simulink model "CSE1_HIL_full16_caseB"  (R2018b)
settings: Solver=VariableStepAuto  StartTime=0.0  StopTime=500  MaxStep=10e-3  RelTol=1e-3
libraries: aerolibutil x1
settings Model: Creator=einarsu  LastModifiedBy=martin
settings OptimizationCC: LifeSpan=inf
settings DebuggingCC: SFExecutionAtInitializationDiag=none
settings SFSimCC: SimUseLocalCustomCode=off
settings RTWCC: RTWUseLocalCustomCode=off
settings CodeAppCC: StateflowObjectComments=on

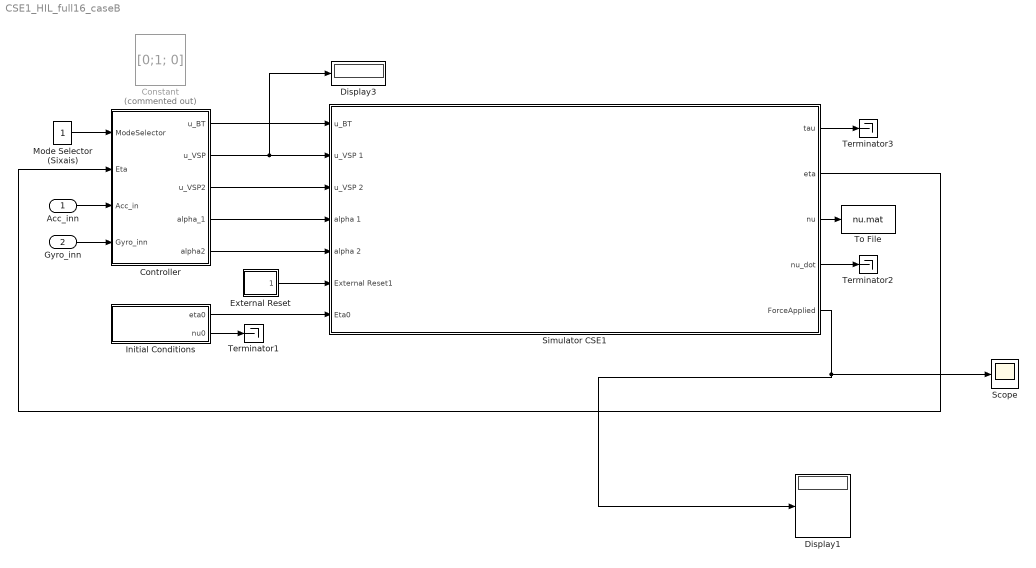
== system CSE1_HIL_full16_caseB ==
  Acc_inn : Inport
  Gyro_inn : Inport  Port=2
  Constant : Constant  Commented=on  Value=[0;1; 0]
  Controller : Subsystem
  Display1 : Display
  Display3 : Display
  External Reset : Subsystem
  "Initial Conditions " : Subsystem
  Mode Selector (Sixais) : Constant
  Scope : Scope
  Simulator CSE1 : Subsystem
  Terminator1 : Terminator
  Terminator2 : Terminator
  Terminator3 : Terminator
  To File : ToFile  Filename=nu.mat  MatrixName=nu
  wires:
  Controller/1(u_BT) -> Simulator CSE1/1(u_BT)
  Controller/4(alpha_1) -> Simulator CSE1/4(alpha 1)
  Controller/2(u_VSP) -> Display3/1, Simulator CSE1/2(u_VSP 1)
  Controller/5(alpha2) -> Simulator CSE1/5(alpha 2)
  Controller/3("u_VSP2 ") -> Simulator CSE1/3(u_VSP 2)
  External Reset/1(Out1) -> Simulator CSE1/6(External Reset1)
  "Initial Conditions "/1(eta0) -> Simulator CSE1/7(Eta0)
  Mode Selector (Sixais)/1 -> Controller/1(ModeSelector)
  Simulator CSE1/2(eta) -> Controller/2(Eta)
  Acc_inn/1 -> Controller/3(Acc_in)
  Gyro_inn/1 -> Controller/4(Gyro_inn)
  Simulator CSE1/5(ForceApplied) -> Scope/1, Display1/1
  "Initial Conditions "/2(nu0) -> Terminator1/1
  Simulator CSE1/4(nu_dot) -> Terminator2/1
  Simulator CSE1/3(nu) -> To File/1
  Simulator CSE1/1(tau) -> Terminator3/1

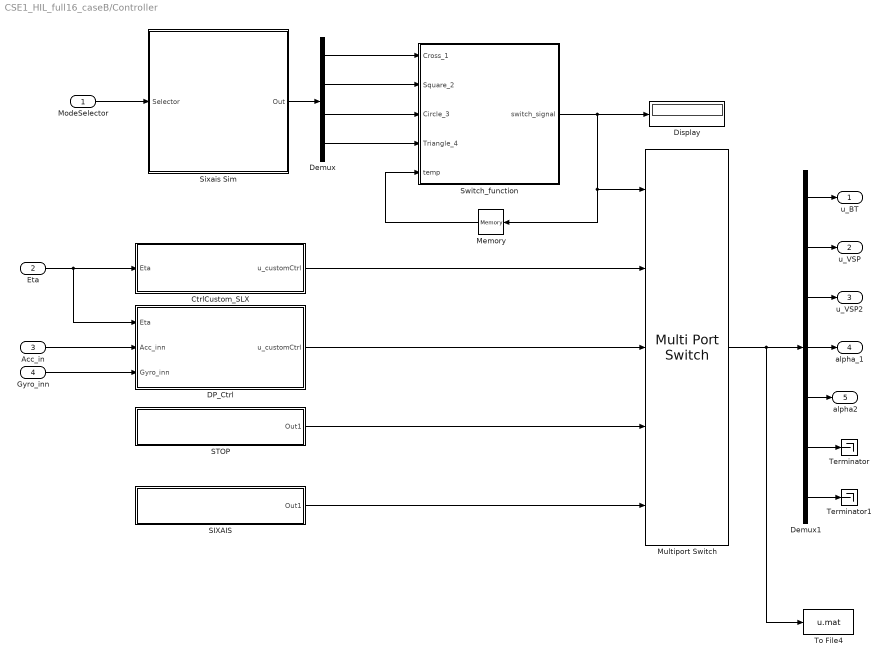
== system CSE1_HIL_full16_caseB/Controller ==
  ModeSelector : Inport
  Eta : Inport  Port=2
  Acc_in : Inport  Port=3
  Gyro_inn : Inport  Port=4
  CtrlCustom_SLX : Subsystem
  DP_Ctrl : Subsystem
  Demux : Demux
  Demux1 : Demux  Outputs=7
  Display : Display
  Memory : Memory  InitialCondition=4
  Multiport Switch : MultiPortSwitch  Inputs=4
  SIXAIS : Subsystem
  STOP : Subsystem
  Sixais Sim : MATLAB Function  TreatAsAtomicUnit=on
  Switch_function : MATLAB Function  TreatAsAtomicUnit=on
  Terminator : Terminator
  Terminator1 : Terminator
  To File4 : ToFile  Filename=u.mat  MatrixName=u
  u_BT : Outport
  u_VSP : Outport  Port=2
  "u_VSP2 " : Outport  Port=3
  alpha_1 : Outport  Port=4
  alpha2 : Outport  Port=5
  wires:
  Memory/1 -> Switch_function/5(temp)
  CtrlCustom_SLX/1(u_customCtrl) -> Multiport Switch/2
  Demux/1 -> Switch_function/1(Cross_1)
  Demux/2 -> Switch_function/2(Square_2)
  Demux/3 -> Switch_function/3(Circle_3)
  Demux/4 -> Switch_function/4(Triangle_4)
  Sixais Sim/1(Out) -> Demux/1
  ModeSelector/1 -> Sixais Sim/1(Selector)
  STOP/1(Out1) -> Multiport Switch/4
  SIXAIS/1(Out1) -> Multiport Switch/5
  Eta/1 -> CtrlCustom_SLX/1(Eta), DP_Ctrl/1(Eta)
  Multiport Switch/1 -> To File4/1, Demux1/1
  Demux1/1 -> u_BT/1
  Demux1/2 -> u_VSP/1
  Demux1/3 -> "u_VSP2 "/1
  Demux1/4 -> alpha_1/1
  Demux1/5 -> alpha2/1
  Demux1/6 -> Terminator/1
  Demux1/7 -> Terminator1/1
  Acc_in/1 -> DP_Ctrl/2(Acc_inn)
  Gyro_inn/1 -> DP_Ctrl/3(Gyro_inn)
  DP_Ctrl/1(u_customCtrl) -> Multiport Switch/3
  Switch_function/1(switch_signal) -> Display/1, Memory/1, Multiport Switch/1

== system CSE1_HIL_full16_caseB/External Reset ==
  note: Most relevant for Real-Time Simulations...
  Constant : Constant  Value=0
  Out1 : Outport
  wires:
  Constant/1 -> Out1/1

== system CSE1_HIL_full16_caseB/Initial Conditions  ==
  Eta0 : Constant  Value=zeros(3,1)
  "V0 " : Constant  Value=zeros(3,1)
  eta0 : Outport
  nu0 : Outport  Port=2
  wires:
  "V0 "/1 -> nu0/1
  Eta0/1 -> eta0/1

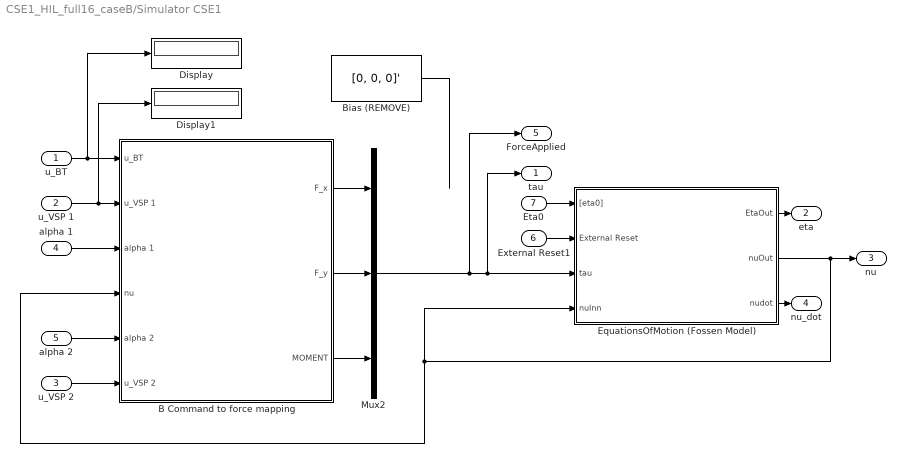
== system CSE1_HIL_full16_caseB/Simulator CSE1 ==
  u_BT : Inport
  u_VSP 1 : Inport  Port=2
  u_VSP 2 : Inport  Port=3
  alpha 1 : Inport  Port=4
  alpha 2 : Inport  Port=5
  External Reset1 : Inport  Port=6
  Eta0 : Inport  Port=7
  B Command to force mapping : Subsystem
  Bias (REMOVE) : Constant  Value=[0, 0, 0]'
  Display : Display
  Display1 : Display
  EquationsOfMotion (Fossen Model) : Subsystem
  Mux2 : Mux  Inputs=3
  tau : Outport
  eta : Outport  Port=2
  nu : Outport  Port=3
  nu_dot : Outport  Port=4
  ForceApplied : Outport  Port=5
  wires:
  alpha 2/1 -> B Command to force mapping/5(alpha 2)
  B Command to force mapping/2("F_y ") -> Mux2/2
  B Command to force mapping/1(F_x) -> Mux2/1
  u_VSP 1/1 -> Display1/1, B Command to force mapping/2(u_VSP 1)
  alpha 1/1 -> B Command to force mapping/3(alpha 1)
  u_BT/1 -> Display/1, B Command to force mapping/1(u_BT)
  u_VSP 2/1 -> B Command to force mapping/6(u_VSP 2)
  EquationsOfMotion (Fossen Model)/2(nuOut) -> B Command to force mapping/4(nu), EquationsOfMotion (Fossen Model)/4(nuInn), nu/1
  Eta0/1 -> EquationsOfMotion (Fossen Model)/1("[eta0] ")
  External Reset1/1 -> EquationsOfMotion (Fossen Model)/2(External Reset)
  EquationsOfMotion (Fossen Model)/1(EtaOut) -> eta/1
  EquationsOfMotion (Fossen Model)/3(nudot) -> nu_dot/1
  B Command to force mapping/3("MOMENT ") -> Mux2/3
  Mux2/1 -> ForceApplied/1, EquationsOfMotion (Fossen Model)/3(tau), tau/1
  Bias (REMOVE)/1 -> ?

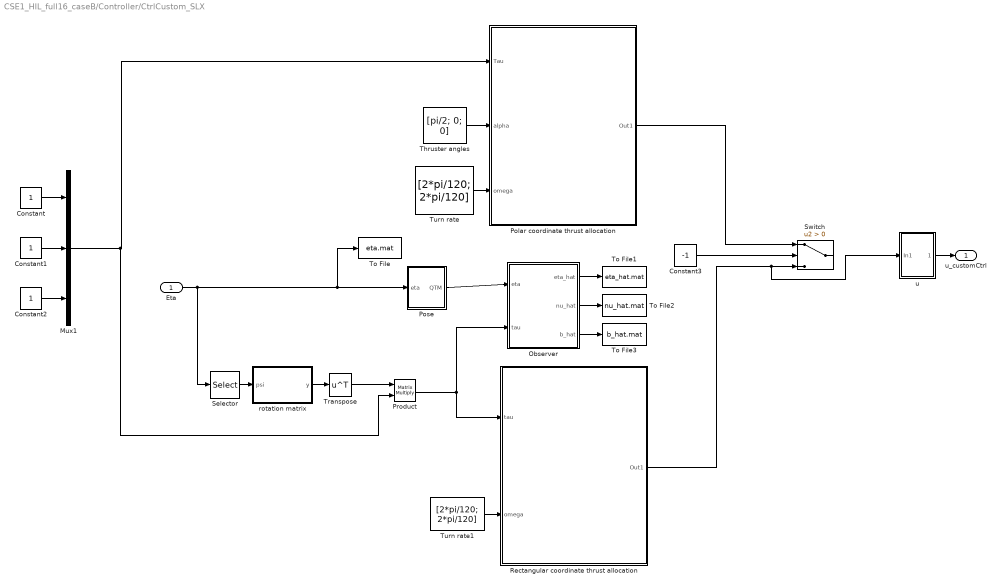
== system CSE1_HIL_full16_caseB/Controller/CtrlCustom_SLX ==
  Eta : Inport
  Constant : Constant
  Constant1 : Constant
  Constant2 : Constant
  Constant3 : Constant  Value=-1
  Mux1 : Mux  Inputs=3
  Observer : Subsystem
  Polar coordinate thrust allocation : Subsystem
  Pose : Subsystem
  Product : Product  Multiplication=Matrix(*)
  Rectangular coordinate thrust allocation : Subsystem
  Selector : Selector  InputPortWidth=3  IndexOptions=Index vector (dialog)  Indices=[3]  OutputSizes=1
  Switch : Switch  Criteria=u2 > Threshold
  Thruster angles : Constant  Value=[pi/2; 0; 0]  VectorParams1D=off
  To File : ToFile  Filename=eta.mat  MatrixName=eta
  To File1 : ToFile  Filename=eta_hat.mat  MatrixName=eta_hat
  To File2 : ToFile  Filename=nu_hat.mat  MatrixName=nu_hat
  To File3 : ToFile  Filename=b_hat.mat  MatrixName=b_hat
  Transpose : Math  Operator=transpose  SaturateOnIntegerOverflow=on
  Turn rate : Constant  Value=[2*pi/120; 2*pi/120]  VectorParams1D=off
  Turn rate1 : Constant  Value=[2*pi/120; 2*pi/120]  VectorParams1D=off
  rotation matrix : MATLAB Function  TreatAsAtomicUnit=on
  u : Subsystem
  u_customCtrl : Outport
  wires:
  Rectangular coordinate thrust allocation/1(Out1) -> u/1(In1), Switch/3
  Turn rate1/1 -> Rectangular coordinate thrust allocation/2("omega ")
  Turn rate/1 -> Polar coordinate thrust allocation/3("omega ")
  Thruster angles/1 -> Polar coordinate thrust allocation/2(alpha)
  Eta/1 -> To File/1, Pose/1(eta), Selector/1
  u/1(Out1) -> u_customCtrl/1
  Polar coordinate thrust allocation/1(Out1) -> Switch/1
  Constant2/1 -> Mux1/3
  Constant1/1 -> Mux1/2
  Constant/1 -> Mux1/1
  Pose/1(QTM) -> Observer/1(eta)
  Mux1/1 -> Product/2, Polar coordinate thrust allocation/1(Tau)
  Observer/1(eta_hat) -> To File1/1
  Observer/2("nu_hat ") -> To File2/1
  Observer/3(b_hat) -> To File3/1
  Constant3/1 -> Switch/2
  Selector/1 -> rotation matrix/1(psi)
  rotation matrix/1(y) -> Transpose/1
  Product/1 -> Observer/2(tau), Rectangular coordinate thrust allocation/1(tau)
  Transpose/1 -> Product/1

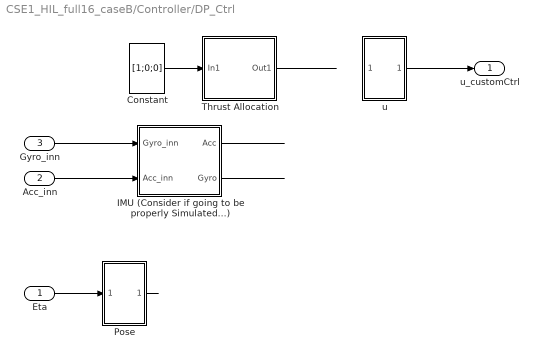
== system CSE1_HIL_full16_caseB/Controller/DP_Ctrl ==
  Eta : Inport
  Acc_inn : Inport  Port=2
  Gyro_inn : Inport  Port=3
  Constant : Constant  Value=[1;0;0]
  IMU (Consider if going to be properly Simulated...) : Subsystem
  Pose : Subsystem
  "Thrust Allocation " : Subsystem
  u : Subsystem
  u_customCtrl : Outport
  wires:
  Pose/1(QTM) -> ?
  Gyro_inn/1 -> IMU (Consider if going to be properly Simulated...)/1(Gyro_inn)
  Acc_inn/1 -> IMU (Consider if going to be properly Simulated...)/2(Acc_inn)
  Eta/1 -> Pose/1(eta)
  u/1(Out1) -> u_customCtrl/1
  IMU (Consider if going to be properly Simulated...)/2(Gyro) -> ?
  IMU (Consider if going to be properly Simulated...)/1(Acc) -> ?
  Constant/1 -> "Thrust Allocation "/1(In1)
  "Thrust Allocation "/1(Out1) -> ?

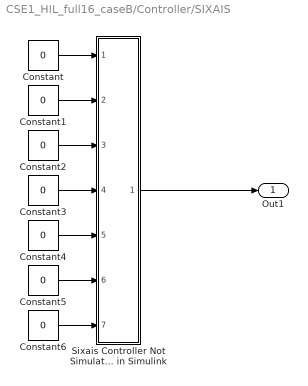
== system CSE1_HIL_full16_caseB/Controller/SIXAIS ==
  Constant{,1..6} (7 alike) : Constant  Value=0
  Sixais Controller Not Simulated in Simulink : Subsystem
  Out1 : Outport
  wires:
  Constant/1 -> Sixais Controller Not Simulated in Simulink/1(In1)
  Constant1/1 -> Sixais Controller Not Simulated in Simulink/2(In2)
  Constant2/1 -> Sixais Controller Not Simulated in Simulink/3(In3)
  Constant3/1 -> Sixais Controller Not Simulated in Simulink/4(In4)
  Constant4/1 -> Sixais Controller Not Simulated in Simulink/5(In5)
  Constant5/1 -> Sixais Controller Not Simulated in Simulink/6(In6)
  Constant6/1 -> Sixais Controller Not Simulated in Simulink/7(In7)
  Sixais Controller Not Simulated in Simulink/1(Out1) -> Out1/1

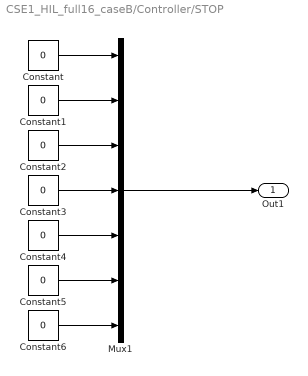
== system CSE1_HIL_full16_caseB/Controller/STOP ==
  Constant{,1..6} (7 alike) : Constant  Value=0
  Mux1 : Mux  Inputs=7
  Out1 : Outport
  wires:
  Mux1/1 -> Out1/1
  Constant/1 -> Mux1/1
  Constant1/1 -> Mux1/2
  Constant2/1 -> Mux1/3
  Constant3/1 -> Mux1/4
  Constant4/1 -> Mux1/5
  Constant5/1 -> Mux1/6
  Constant6/1 -> Mux1/7

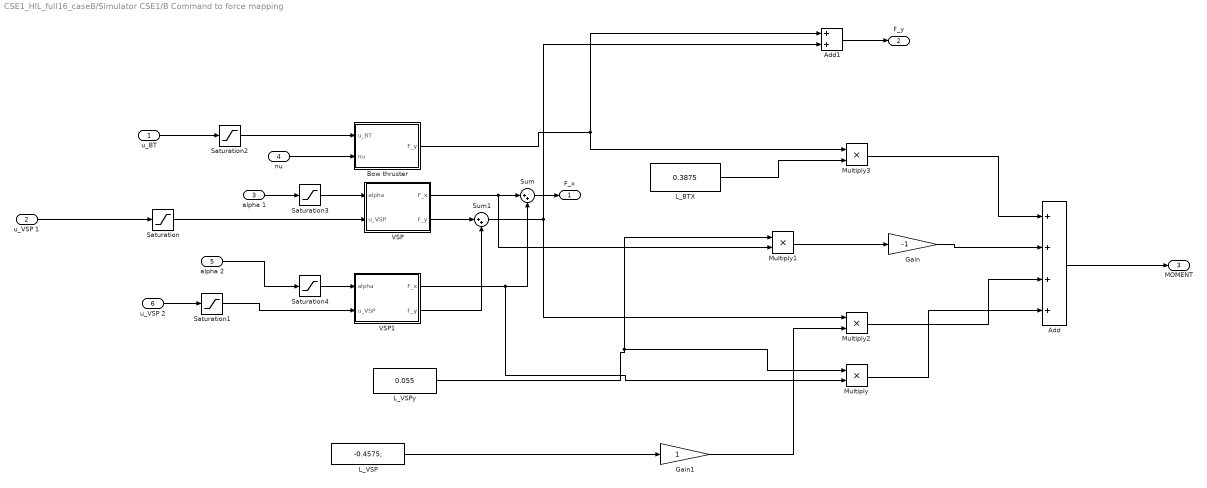
== system CSE1_HIL_full16_caseB/Simulator CSE1/B Command to force mapping ==
  u_BT : Inport
  u_VSP 1 : Inport  Port=2
  alpha 1 : Inport  Port=3
  nu : Inport  Port=4
  alpha 2 : Inport  Port=5
  u_VSP 2 : Inport  Port=6
  Add : Sum  Inputs=++++
  Add1 : Sum
  Bow thruster : MATLAB Function  TreatAsAtomicUnit=on
  Gain : Gain  Gain=-1
  Gain1 : Gain
  L_BTX : Constant  Value=0.3875
  L_VSP : Constant  Value=-0.4575;
  L_VSPy : Constant  Value=0.055
  Multiply{,1..3} (4 alike) : Product
  Saturation : Saturate  UpperLimit=1  LowerLimit=0
  Saturation1 : Saturate  UpperLimit=1  LowerLimit=0
  Saturation2 : Saturate  UpperLimit=1  LowerLimit=-1
  Saturation3 : Saturate  UpperLimit=pi  LowerLimit=-pi
  Saturation4 : Saturate  UpperLimit=pi  LowerLimit=-pi
  Sum : Sum  Inputs=|++
  Sum1 : Sum  Inputs=|++
  VSP : MATLAB Function  TreatAsAtomicUnit=on
  VSP1 : MATLAB Function  TreatAsAtomicUnit=on
  F_x : Outport
  "F_y " : Outport  Port=2
  "MOMENT " : Outport  Port=3
  wires:
  alpha 1/1 -> Saturation3/1
  nu/1 -> Bow thruster/2(nu)
  Bow thruster/1(F_y) -> Add1/1, Multiply3/1
  VSP/2(F_y) -> Sum1/1
  Sum1/1 -> Add1/2, Multiply2/1
  VSP1/2(F_y) -> Sum1/2
  VSP1/1(F_x) -> Multiply/2, Sum/2
  VSP/1(F_x) -> Multiply1/2, Sum/1
  Sum/1 -> F_x/1
  alpha 2/1 -> Saturation4/1
  u_VSP 2/1 -> Saturation1/1
  L_VSP/1 -> Gain1/1
  L_BTX/1 -> Multiply3/2
  L_VSPy/1 -> Multiply/1, Multiply1/1
  Multiply3/1 -> Add/1
  Multiply1/1 -> Gain/1
  Multiply2/1 -> Add/3
  Multiply/1 -> Add/4
  Add/1 -> "MOMENT "/1
  Gain/1 -> Add/2
  Gain1/1 -> Multiply2/2
  Add1/1 -> "F_y "/1
  Saturation/1 -> VSP/2(u_VSP)
  Saturation1/1 -> VSP1/2(u_VSP)
  u_BT/1 -> Saturation2/1
  u_VSP 1/1 -> Saturation/1
  Saturation2/1 -> Bow thruster/1(u_BT)
  Saturation3/1 -> VSP/1(alpha)
  Saturation4/1 -> VSP1/1(alpha)

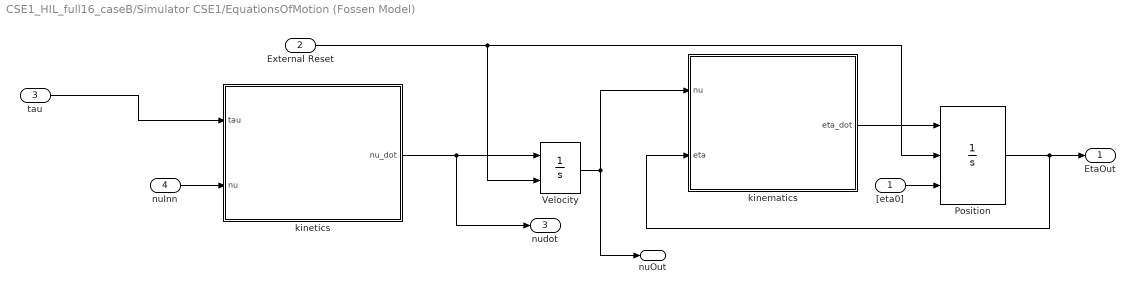
== system CSE1_HIL_full16_caseB/Simulator CSE1/EquationsOfMotion (Fossen Model) ==
  "[eta0] " : Inport
  External Reset : Inport  Port=2
  tau : Inport  Port=3
  nuInn : Inport  Port=4
  Position : Integrator  ExternalReset=either  InitialConditionSource=external  InitialCondition=[0 0 0]'
  Velocity : Integrator  ExternalReset=either  InitialCondition=[0 0 0]'
  kinematics : MATLAB Function  TreatAsAtomicUnit=on
  kinetics : MATLAB Function  TreatAsAtomicUnit=on
  EtaOut : Outport
  nuOut : Outport  Port=2
  nudot : Outport  Port=3
  wires:
  tau/1 -> kinetics/1(tau)
  Position/1 -> kinematics/2(eta), EtaOut/1
  "[eta0] "/1 -> Position/3
  nuInn/1 -> kinetics/2(nu)
  kinematics/1(eta_dot) -> Position/1
  Velocity/1 -> kinematics/1(nu), nuOut/1
  kinetics/1(nu_dot) -> nudot/1, Velocity/1
  External Reset/1 -> Position/2, Velocity/2

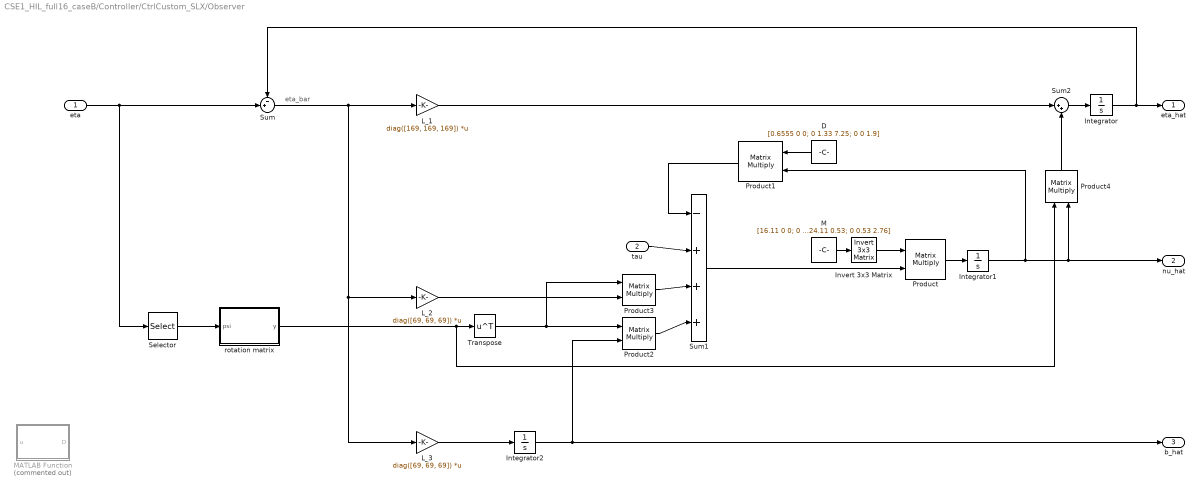
== system CSE1_HIL_full16_caseB/Controller/CtrlCustom_SLX/Observer ==
  note: eta_bar
  eta : Inport
  tau : Inport  Port=2
  D : Constant  Value=[0.6555 0 0; 0 1.33 7.25; 0 0 1.9]
  Integrator : Integrator  InitialCondition=[0 0 0]'
  Integrator1 : Integrator  InitialCondition=[0 0 0]'
  Integrator2 : Integrator
  Invert 3x3 Matrix : aerolibutil/Invert  3x3 Matrix
  L_1 : Gain  Gain=diag([169, 169, 169])  Multiplication=Matrix(K*u)
  L_2 : Gain  Gain=diag([69, 69, 69])  Multiplication=Matrix(K*u)
  L_3 : Gain  Gain=diag([69, 69, 69])  Multiplication=Matrix(K*u)
  M : Constant  Value=[16.11 0 0; 0 24.11 0.53; 0 0.53 2.76]
  MATLAB Function : MATLAB Function  Commented=on  TreatAsAtomicUnit=on
  Product{,1..4} (5 alike) : Product  Multiplication=Matrix(*)
  Selector : Selector  InputPortWidth=3  IndexOptions=Index vector (dialog)  Indices=[3]  OutputSizes=1
  Sum : Sum  Inputs=-+|
  Sum1 : Sum  Inputs=-|+|+|+
  Sum2 : Sum  Inputs=|++
  Transpose : Math  Operator=transpose  SaturateOnIntegerOverflow=on
  rotation matrix : MATLAB Function  TreatAsAtomicUnit=on
  eta_hat : Outport
  "nu_hat " : Outport  Port=2
  b_hat : Outport  Port=3
  wires:
  Sum/1 -> L_3/1, L_2/1, L_1/1
  eta/1 -> Selector/1, Sum/2
  Selector/1 -> rotation matrix/1(psi)
  Integrator/1 -> eta_hat/1, Sum/1
  Invert 3x3 Matrix/1 -> Product/1
  M/1 -> Invert 3x3 Matrix/1
  D/1 -> Product1/1
  Product1/1 -> Sum1/1
  rotation matrix/1(y) -> Product4/1, Transpose/1
  Transpose/1 -> Product3/1, Product2/1
  L_2/1 -> Product3/2
  Sum1/1 -> Product/2
  Product/1 -> Integrator1/1
  L_1/1 -> Sum2/1
  Product4/1 -> Sum2/2
  Sum2/1 -> Integrator/1
  Integrator1/1 -> Product1/2, Product4/2, "nu_hat "/1
  L_3/1 -> Integrator2/1
  Integrator2/1 -> Product2/2, b_hat/1
  Product2/1 -> Sum1/4
  Product3/1 -> Sum1/3
  tau/1 -> Sum1/2

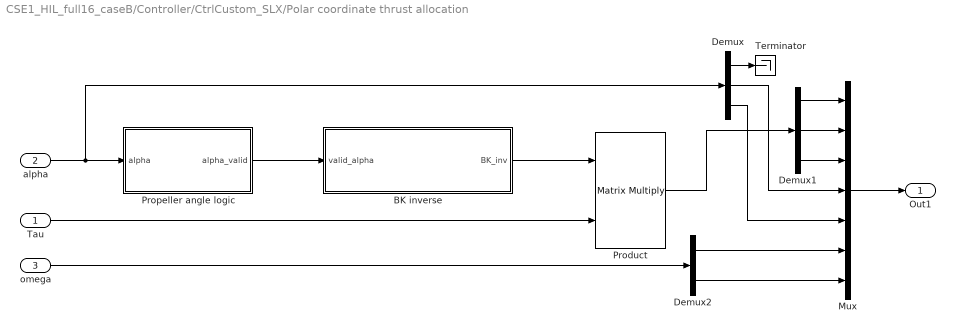
== system CSE1_HIL_full16_caseB/Controller/CtrlCustom_SLX/Polar coordinate thrust allocation ==
  Tau : Inport
  alpha : Inport  Port=2
  "omega " : Inport  Port=3
  "BK inverse " : MATLAB Function  TreatAsAtomicUnit=on
  Demux : Demux  Outputs=3
  Demux1 : Demux  Outputs=3
  Demux2 : Demux  Outputs=2
  Mux : Mux  Inputs=7
  Product : Product  Multiplication=Matrix(*)
  Propeller angle logic : MATLAB Function  TreatAsAtomicUnit=on
  Terminator : Terminator
  Out1 : Outport
  wires:
  Demux2/2 -> Mux/7
  Demux2/1 -> Mux/6
  Product/1 -> Demux1/1
  Demux1/3 -> Mux/3
  Demux1/2 -> Mux/2
  Demux1/1 -> Mux/1
  Demux/3 -> Mux/5
  Demux/2 -> Mux/4
  Demux/1 -> Terminator/1
  Mux/1 -> Out1/1
  "omega "/1 -> Demux2/1
  Tau/1 -> Product/2
  "BK inverse "/1(BK_inv) -> Product/1
  Propeller angle logic/1(alpha_valid) -> "BK inverse "/1(valid_alpha)
  alpha/1 -> Propeller angle logic/1(alpha), Demux/1

== system CSE1_HIL_full16_caseB/Controller/CtrlCustom_SLX/Pose ==
  eta : Inport
  Demux : Demux  Outputs=3
  Mux : Mux  Inputs=3
  QTM : Outport
  wires:
  eta/1 -> Demux/1
  Mux/1 -> QTM/1
  Demux/1 -> Mux/1  "x_m"
  Demux/3 -> Mux/3  "psi_m"
  Demux/2 -> Mux/2  "y_m"

== system CSE1_HIL_full16_caseB/Controller/CtrlCustom_SLX/Rectangular coordinate thrust allocation ==
  tau : Inport
  "omega " : Inport  Port=2
  Demux : Demux  Outputs=5
  Demux1 : Demux  Outputs=2
  MATLAB Function : MATLAB Function  TreatAsAtomicUnit=on
  Mux : Mux  Inputs=7
  Selector : Selector  InputPortWidth=5  IndexOptions=Index vector (dialog)  Indices=[3 1 2 4 5]  OutputSizes=1
  Out1 : Outport
  wires:
  Mux/1 -> Out1/1
  Demux1/1 -> Mux/6
  Demux1/2 -> Mux/7
  Demux/5 -> Mux/5
  Demux/4 -> Mux/4
  "omega "/1 -> Demux1/1
  MATLAB Function/1(u_ext) -> Selector/1
  tau/1 -> MATLAB Function/1(tau)
  Demux/1 -> Mux/1
  Demux/2 -> Mux/2
  Demux/3 -> Mux/3
  Selector/1 -> Demux/1

== system CSE1_HIL_full16_caseB/Controller/CtrlCustom_SLX/u ==
  In1 : Inport
  Demux1 : Demux  Outputs=7
  Mux : Mux  Inputs=7
  Saturation1 : Saturate  UpperLimit=1  LowerLimit=0
  Saturation11 : Saturate  UpperLimit=1  LowerLimit=0
  Saturation2 : Saturate  UpperLimit=1  LowerLimit=-1
  Out1 : Outport
  wires:
  Saturation1/1 -> Mux/3
  Saturation11/1 -> Mux/2
  Mux/1 -> Out1/1
  Demux1/7 -> Mux/7  "omega_VSP2"
  Demux1/6 -> Mux/6  "omega_VSP1"
  Demux1/5 -> Mux/5  "alpha_VSP2"
  Demux1/4 -> Mux/4  "alpha_VSP1"
  Demux1/3 -> Saturation1/1  "u_VSP2"
  Demux1/2 -> Saturation11/1  "u_VSP1"
  Demux1/1 -> Saturation2/1  "u_BT"
  In1/1 -> Demux1/1
  Saturation2/1 -> Mux/1

== system CSE1_HIL_full16_caseB/Controller/DP_Ctrl/IMU (Consider if going to be properly Simulated...) ==
  Gyro_inn : Inport
  Acc_inn : Inport  Port=2
  Demux : Demux  Outputs=3
  Demux1 : Demux  Outputs=3
  Mux : Mux  Inputs=3
  Mux2 : Mux  Inputs=3
  Acc : Outport
  Gyro : Outport  Port=2
  wires:
  Acc_inn/1 -> Demux1/1
  Gyro_inn/1 -> Demux/1
  Demux/1 -> Mux2/1
  Demux/2 -> Mux2/2
  Demux/3 -> Mux2/3
  Demux1/2 -> Mux/2
  Demux1/3 -> Mux/3
  Mux2/1 -> Gyro/1
  Demux1/1 -> Mux/1
  Mux/1 -> Acc/1

== system CSE1_HIL_full16_caseB/Controller/DP_Ctrl/Pose ==
  eta : Inport
  Demux : Demux  Outputs=3
  Mux : Mux  Inputs=3
  QTM : Outport
  wires:
  eta/1 -> Demux/1
  Mux/1 -> QTM/1
  Demux/1 -> Mux/1  "x_m"
  Demux/3 -> Mux/3  "psi_m"
  Demux/2 -> Mux/2  "y_m"

== system CSE1_HIL_full16_caseB/Controller/DP_Ctrl/Thrust Allocation  ==
  In1 : Inport
  THALOC (u->tau) : MATLAB Function  TreatAsAtomicUnit=on
  Out1 : Outport
  wires:
  In1/1 -> THALOC (u->tau)/1(u)
  THALOC (u->tau)/1(y) -> Out1/1

== system CSE1_HIL_full16_caseB/Controller/DP_Ctrl/u ==
  In1 : Inport
  Demux1 : Demux  Outputs=7
  Mux : Mux  Inputs=7
  Out1 : Outport
  wires:
  Mux/1 -> Out1/1
  Demux1/7 -> Mux/7  "omega_VSP2"
  Demux1/6 -> Mux/6  "omega_VSP1"
  Demux1/5 -> Mux/5  "alpha_VSP2"
  Demux1/4 -> Mux/4  "alpha_VSP1"
  Demux1/3 -> Mux/3  "u_VSP2"
  Demux1/2 -> Mux/2  "u_VSP1"
  Demux1/1 -> Mux/1  "u_BT"
  In1/1 -> Demux1/1

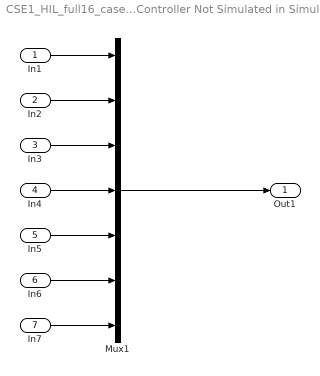
== system CSE1_HIL_full16_caseB/Controller/SIXAIS/Sixais Controller Not Simulated in Simulink ==
  In1 : Inport
  In2 : Inport  Port=2
  In3 : Inport  Port=3
  In4 : Inport  Port=4
  In5 : Inport  Port=5
  In6 : Inport  Port=6
  In7 : Inport  Port=7
  Mux1 : Mux  Inputs=7
  Out1 : Outport
  wires:
  In4/1 -> Mux1/4
  In5/1 -> Mux1/5
  In6/1 -> Mux1/6
  In3/1 -> Mux1/3
  In1/1 -> Mux1/1
  In2/1 -> Mux1/2
  Mux1/1 -> Out1/1
  In7/1 -> Mux1/7

== matlab function CSE1_HIL_full16_caseB/Simulator CSE1/EquationsOfMotion (Fossen Model)/kinematics ==
  data: nu input; eta_dot output; eta input
function eta_dot = CSE1_eta_dot(nu,eta)

psi = eta(3);

J = [cos(psi) -sin(psi) 0
     sin(psi) cos(psi)  0
     0        0         1];

eta_dot = J*nu;

== matlab function CSE1_HIL_full16_caseB/Simulator CSE1/EquationsOfMotion (Fossen Model)/kinetics ==
  data: tau input; nu_dot output; nu input
function nu_dot = CSE1_nu_dot(tau,nu)

u   = nu(1);
v   = nu(2);
r   = nu(3);

tau = [tau(1);tau(2);tau(3)];
%% MATRICES 
%changed m from 14.79 to 14.11

m    = 14.11;   I_z  =  1.7600;   x_g = 0.0375;       % x_g  =  0.0460; % Table B.1

%% Added mass
%changed Y_vd from -1.0 to -10.0
X_ud  =     -2.0;											% Table B.1
					Y_vd =      -10.0;	N_vd =    -0.0;		% Table B.1
					Y_rd =      -0.0;	N_rd =    -1.0;		% Table B.1

%% Total mass matrix
m_11 = m-X_ud;
m_22 = m-Y_vd;
m_23 = m*x_g-Y_rd;
m_32 = m*x_g-N_vd; % noted as Y_rd in handbook, but same value
m_33 = I_z-N_rd;

M    = [m_11 0    0
        0    m_22 m_23
        0    m_32 m_33];
	
%% Damping coefficients
% Comments at the end of the lines indicate the old values used.
X_u		= -0.6555;		X_v		= 0;
X_uu 	= 0.3545;		X_vv	= -2.443;
X_uuu 	= -3.787;		X_vvv	= 0;

						Y_v		= -1.33; 			Y_r		= -7.250; % Y_r
						Y_vv	= -2.776;			Y_rr	= -3.450; % Y_rr
						Y_vvv	= -64.91;			Y_rrr	= 0;
						
						Y_rv	= -0.805;			Y_vr	= -0.845; % Y_rv, Y_vr

						N_v		= 0;				N_r		= -1.900; % N_r
						N_vv	= -0.2088;			N_rr	= -0.750; % N_rr
						N_vvv	= 0;				N_rrr	= 0;
						
						N_rv	= 0.130;			N_vr	= 0.080; % N_rv, N_vr

%% Correolis matrix
c_13 = -(m-Y_vd)*v-(m*x_g-Y_rd)*r;
c_23 = (m-X_ud)*u;
C    = [0     0     c_13
        0     0     c_23
        -c_13 -c_23 0   ];

%% Assembly of the damping matrix
%should be abs(u), abs(v) some places, only positive values? 

d_11 = -X_u - X_uu*u - X_uuu*u^2;
d_22 = -Y_v - Y_vv*v - Y_vvv*v^2 - Y_rv*abs(r);
d_33 = -N_r - N_rr*abs(r) - N_rrr*r^2 - N_vr*abs(v); % using abs(r)

d_12 = -X_v - X_vv*v - X_vvv*v^2;
d_23 = -Y_r - Y_rr*abs(r) - Y_rrr*r^2 - Y_vr*abs(v);
d_32 = -N_v - N_vv*v - N_vvv*v^2 - N_rv*abs(r);

%D    = [d_11 d_12 0      vet ikke hvorfor d_12 er her
%        0    d_22 d_23
%        0    d_32 d_33];
D    = [d_11 0 0
        0    d_22 d_23
        0    d_32 d_33];


%% CALCULATION
nu_dot = M\(tau-(C+D)*nu);

== matlab function CSE1_HIL_full16_caseB/Controller/CtrlCustom_SLX/Polar coordinate thrust allocation/Propeller angle logic ==
  data: alpha input; alpha_valid output
function alpha_valid = fcn(alpha)

%Propeller 1

if alpha(2) > pi
    alpha(2) = pi;
elseif alpha(2) < -pi
    alpha(2) = -pi;
end
    
%Propeller 2

if alpha(3) > pi
    alpha(3) = pi;
elseif alpha(3) < -pi
    alpha(3) = -pi;
end

alpha(1) = pi/2;
    
alpha_valid = alpha;

== matlab function CSE1_HIL_full16_caseB/Controller/CtrlCustom_SLX/Polar coordinate thrust allocation/BK inverse  ==
  data: valid_alpha input; BK_inv output
function BK_inv = fcn(valid_alpha)

k_1 = 2.629;
k_2 = 1.03;
k_3 = 1.03;

K = diag([k_1, k_2, k_3]);

alpha_1 = valid_alpha(1);
alpha_2 = valid_alpha(2);
alpha_3 = valid_alpha(3);

L_xvsp = 0.4574;
L_yvsp = 0.055;
L_bt = 0.3875;

L_xvsp_1 = -L_xvsp;
L_yvsp_1 = -L_yvsp;
L_xvsp_2 = -L_xvsp;
L_yvsp_2 = L_yvsp;

B = [0, cos(alpha_2), cos(alpha_3);
     1, sin(alpha_2), sin(alpha_3);
     L_bt, -L_yvsp_1*cos(alpha_2) + L_xvsp_1*sin(alpha_2), -L_yvsp_2*cos(alpha_3) ...
     + L_xvsp_2*sin(alpha_3)];
 
BK = B*K;

BK_inv = pinv(BK);

== matlab function CSE1_HIL_full16_caseB/Controller/CtrlCustom_SLX/Rectangular coordinate thrust allocation/MATLAB Function ==
  data: tau input; u_ext output
function u_ext = fcn(tau)

%%
%Initialize extended thrust allocation matrix
L_xvsp = 0.4574;
L_yvsp = 0.055;
L_bt = 0.3875;

L_xvsp_1 = -L_xvsp;
L_yvsp_1 = -L_yvsp;
L_xvsp_2 = -L_xvsp;
L_yvsp_2 = L_yvsp;

B_ext = [1         0        1         0        0;
         0         1        0         1        1;
        -L_yvsp_1  L_xvsp_1 -L_yvsp_2 L_xvsp_2 L_bt];
 
B_ext_inv = pinv(B_ext);

%Extended force vector
f = B_ext_inv*tau;

%%
%Calculate angles and control input
alpha_1 = atan2(f(2), f(1));
alpha_2 = atan2(f(4), f(3));

alpha = [alpha_1; alpha_2];

k_1 = 2.629;
k_2 = 1.03;
k_3 = 1.03;

u_1 = (1/k_2)*sqrt(f(1)^2 + f(2)^2);
u_2 = (1/k_3)*sqrt(f(3)^2 + f(4)^2);
u_3 = f(5)/k_1;

u = [u_1; u_2; u_3];

u_ext = [u; alpha];

== matlab function CSE1_HIL_full16_caseB/Controller/CtrlCustom_SLX/rotation matrix ==
  data: psi input; y output
function y = rotation_matrix(psi)

y = [cos(psi) -sin(psi) 0;
    sin(psi) cos(psi) 0;
    0 0 1];
 end

== matlab function CSE1_HIL_full16_caseB/Controller/CtrlCustom_SLX/Observer/rotation matrix ==
  data: psi input; y output
function y = rotation_matrix(psi)

y = [cos(psi) -sin(psi) 0;
    sin(psi) cos(psi) 0;
    0 0 1];
 end

== matlab function CSE1_HIL_full16_caseB/Controller/Switch_function ==
  data: Cross_1 input; switch_signal output; Square_2 input; Circle_3 input; Triangle_4 input; temp input
%% Function that takes in impulse button sigals [0,1] and sends out a 
% different signal depentent pn which button has been pressed

function switch_signal = fcn(Cross_1,Square_2,Circle_3,Triangle_4,temp)
%#codegen
persistent signal;

signal = temp;

if Cross_1 ~= 0
    signal = 1;
end

if Square_2 ~= 0
    signal = 2;
end

if Circle_3 ~= 0
    signal = 3;
end
    
if Triangle_4 ~= 0
    signal = 4; 
end

switch_signal = signal;

== matlab function CSE1_HIL_full16_caseB/Controller/Sixais Sim ==
  data: Selector input; Out output
%% Function that takes in impulse button sigals [0,1] and sends out a 
% different signal depentent pn which button has been pressed

function Out = fcn(Selector)
%#codegen
if Selector==1
    Out=[1 0 0 0];
elseif Selector==2
        Out=[0 1 0 0];
elseif Selector==4
        Out=[0 0 0 1];
else 
        Out=[0 0 1 0];

end

== matlab function CSE1_HIL_full16_caseB/Controller/DP_Ctrl/Thrust Allocation /THALOC (u->tau) ==
  data: u input; y output
function y = fcn(u)

y = u;

== matlab function CSE1_HIL_full16_caseB/Controller/CtrlCustom_SLX/Observer/MATLAB Function ==
  data: u input; D output
function D = fcn(u)

d11 = 0.6555;   %% - 0.3545*sqrt(u(1)^2) + 3.787*u(1)^2;
d22 = 1.33;     %% + 2.776*sqrt(u(2)^2) + 64.91*u(2)^2 + 0.805*sqrt(u(2)^2);
d23 = 7.25;     %% + 0.845*sqrt(u(2)^2) +3.45*sqrt(u(3)^2);
d32 = 0;        %%0.2088*sqrt(u(2)^2) - 0.130*sqrt(u(3)^2);
d33 = 1.9;      % - 0.080*sqrt(u(3)^2) + 0.75*sqrt(u(3)^2);

D = [d11    0       0;
     0      d22     d23;
     0      d32     d33];

== matlab function CSE1_HIL_full16_caseB/Simulator CSE1/B Command to force mapping/Bow thruster ==
  data: u_BT input; F_y output; nu input
function F_y = fcn(u_BT,nu)
%#codegen
u = nu(1);
% Thruster characteristics
if u_BT >0
    u_BT=u_BT+ 0.059;
    a =        -548;
    b =       0.193;
    c =       548.2;
    d =      0.1992;
    y0 = -(a*exp(b*-u_BT) + c*exp(d*-u_BT));
elseif u_BT < 0
    u_BT=u_BT- 0.059;
    a =        -548;
    b =       0.193;
    c =       548.2;
    d =      0.1992;
    y0 = a*exp(b*u_BT) + c*exp(d*u_BT);
else
    y0 = 0;
end
% Thruster losses due to forward speed
a0 =      0.7561;
a1 =      0.3075;
b1 =      -10.22;
c1 =       2.947;
F_y = y0*(a0 + a1*atan(b1*u +c1))/1.1385;
F_y=F_y*2.62/2.7629;


%2019 changes- Some add-hock changes, because it did not make sense previously.

== matlab function CSE1_HIL_full16_caseB/Simulator CSE1/B Command to force mapping/VSP ==
  data: alpha input; F_x output; u_VSP input; F_y output
function [ F_x , F_y ] = fcn(alpha,u_VSP)
%#codegen
% Calculating the force in x-direction
a1 =       1.107  ;
b1 =       1.001  ;
c1 =       1.564  ;
a2 =      0.3471 ;
b2 =      0.1397 ;
c2 =      -1.599  ;
a3 =      0.1558 ;
b3 =       1.993  ;
c3 =       1.886  ;
a4 =      0.1599 ;
b4 =       0.218  ;
c4 =       1.513  ;
a5 =     0.08237 ;
b5 =       2.986  ;
c5 =      -1.601  ;
a6 =     0.04641 ;
b6 =       3.964  ;
c6 =       1.738  ;
F_x =   u_VSP*( a1*sin(b1*alpha+c1) + ...
                a2*sin(b2*alpha+c2) + ...
                a3*sin(b3*alpha+c3) + ...
                a4*sin(b4*alpha+c4) + ...
                a5*sin(b5*alpha+c5) + ...
                a6*sin(b6*alpha+c6) );
% Calculating the force in y-direction
a1 =      0.7936 ;
b1 =       1.001  ;
c1 =     0.01605;
a2 =      0.2112 ;
b2 =       1.997  ;
c2 =     0.03229;
a3 =     0.07608;
b3 =       2.991  ;
c3 =       2.986  ;
a4 =     0.04817;
b4 =       3.999  ;
c4 =     -0.8668 ;
a5 =     0.01757;
b5 =       4.904  ;
c5 =      -2.622 ;
a6 =    -0.02089;
b6 =       5.068  ;
c6 =      0.2548 ;
F_y =   u_VSP*( a1*sin(b1*alpha+c1) + ...
                a2*sin(b2*alpha+c2) + ...
                a3*sin(b3*alpha+c3) + ...
                a4*sin(b4*alpha+c4) + ...
                a5*sin(b5*alpha+c5) + ...
                a6*sin(b6*alpha+c6));

== matlab function CSE1_HIL_full16_caseB/Simulator CSE1/B Command to force mapping/VSP1 ==
  data: alpha input; F_x output; u_VSP input; F_y output
function [ F_x , F_y ] = fcn(alpha,u_VSP)
%#codegen
% Calculating the force in x-direction
a1 =       1.107  ;
b1 =       1.001  ;
c1 =       1.564  ;
a2 =      0.3471 ;
b2 =      0.1397 ;
c2 =      -1.599  ;
a3 =      0.1558 ;
b3 =       1.993  ;
c3 =       1.886  ;
a4 =      0.1599 ;
b4 =       0.218  ;
c4 =       1.513  ;
a5 =     0.08237 ;
b5 =       2.986  ;
c5 =      -1.601  ;
a6 =     0.04641 ;
b6 =       3.964  ;
c6 =       1.738  ;
F_x =   u_VSP*( a1*sin(b1*alpha+c1) + ...
                a2*sin(b2*alpha+c2) + ...
                a3*sin(b3*alpha+c3) + ...
                a4*sin(b4*alpha+c4) + ...
                a5*sin(b5*alpha+c5) + ...
                a6*sin(b6*alpha+c6) );
% Calculating the force in y-direction
a1 =      0.7936 ;
b1 =       1.001  ;
c1 =     0.01605;
a2 =      0.2112 ;
b2 =       1.997  ;
c2 =     0.03229;
a3 =     0.07608;
b3 =       2.991  ;
c3 =       2.986  ;
a4 =     0.04817;
b4 =       3.999  ;
c4 =     -0.8668 ;
a5 =     0.01757;
b5 =       4.904  ;
c5 =      -2.622 ;
a6 =    -0.02089;
b6 =       5.068  ;
c6 =      0.2548 ;
F_y =   u_VSP*( a1*sin(b1*alpha+c1) + ...
                a2*sin(b2*alpha+c2) + ...
                a3*sin(b3*alpha+c3) + ...
                a4*sin(b4*alpha+c4) + ...
                a5*sin(b5*alpha+c5) + ...
                a6*sin(b6*alpha+c6));
